simulink model "RL_sus_quarter_sim"  (R2025a)
settings: Solver=FixedStepAuto  StartTime=0.0  StopTime=20  FixedStep=0.001  RelTol=1e-3
model workspace (MAT data in the model file):
  G0 : Simulink.Parameter (value not decoded)
  Q_F : Simulink.Parameter (value not decoded)
  Q_dot_s : Simulink.Parameter (value not decoded)
  Q_dot_s_h : Simulink.Parameter (value not decoded)
  Q_dot_u : Simulink.Parameter (value not decoded)
  Q_flec : Simulink.Parameter (value not decoded)
  Q_flec_t : Simulink.Parameter (value not decoded)
  b_deflec : Simulink.Parameter (value not decoded)
  bump_height : Simulink.Parameter (value not decoded)
  bump_lenth : Simulink.Parameter (value not decoded)
  bump_start : Simulink.Parameter (value not decoded)
  f0 : Simulink.Parameter (value not decoded)
  kt : Simulink.Parameter (value not decoded)
  ms : Simulink.Parameter (value not decoded)
  n0 : Simulink.Parameter (value not decoded)
  n1 : Simulink.Parameter (value not decoded)
  omega_1 : Simulink.Parameter (value not decoded)
  omega_2 : Simulink.Parameter (value not decoded)
  omega_3 : Simulink.Parameter (value not decoded)
  omega_4 : Simulink.Parameter (value not decoded)
  ramp_height : Simulink.Parameter (value not decoded)
  ramp_lenth : Simulink.Parameter (value not decoded)
  ramp_start : Simulink.Parameter (value not decoded)
  sine_amp : Simulink.Parameter (value not decoded)
  sine_freq : Simulink.Parameter (value not decoded)
  u : Simulink.Parameter (value not decoded)
symbols that are objects in the model workspace (value not decoded): b_deflec, bump_height, bump_lenth, bump_start, f0, G0, kt, ms, n0, n1, omega_1, omega_2, omega_3, omega_4, Q_dot_s, Q_dot_s_h, Q_F, Q_flec, Q_flec_t, ramp_height, ramp_lenth, ramp_start, sine_amp, sine_freq
undefined symbols (not defined in the file): Ground, Hook, SH_ADD_new_as_as_xdef
libraries: fl_lib x250, nesl_utility x48, sharedTrackingLibrary x34, dspstat3 x18, simulink x3, deeplib x2, slpidlib x1
(part 4 of 12)

== system RL_sus_quarter_sim/road_profile/origin ==
  Radio Button : RadioButtonGroup  LabelPosition=Hide  SelectedLabel=随机路面  ButtonGroupName=Group
  road_profile : Subsystem
  路面选择 : Constant  Value=3  OutDataTypeStr=int8
  "Road " : Outport
  wires:
  road_profile/1("Road ") -> "Road "/1  "Zr"
  路面选择/1 -> road_profile/1(Road_selection)

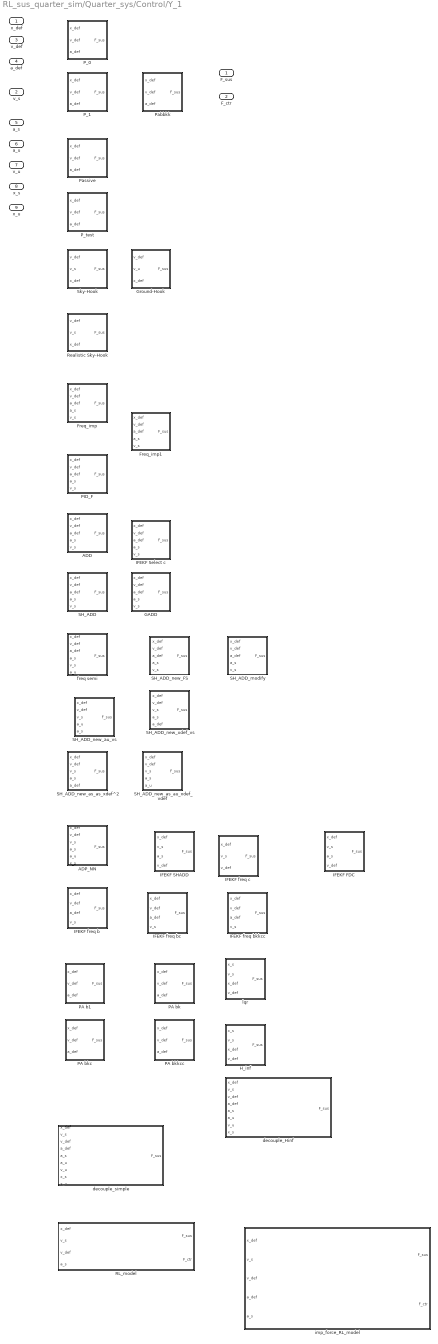
== system RL_sus_quarter_sim/Quarter_sys/Control/Y_1 ==
  x_def : Inport
  v_s : Inport  Port=2
  v_def : Inport  Port=3
  a_def : Inport  Port=4
  a_s : Inport  Port=5
  a_u : Inport  Port=6
  v_u : Inport  Port=7
  x_s : Inport  Port=8
  x_u : Inport  Port=9
  ADD : Subsystem  VariantControl=ADD
  ADP_NN : Subsystem  VariantControl=ADP_nn
  Freq_imp : Subsystem  VariantControl=Freq_Impedance
  Freq_imp1 : Subsystem  VariantControl=Freq_imp1
  GADD : Subsystem  VariantControl=GADD
  Ground-Hook : Subsystem  VariantControl=Ground-Hook
  H_inf : Subsystem  VariantControl=H_inf
  IFEKF FDC : Subsystem  VariantControl=IFEKF FDC
  IFEKF SHADD : Subsystem  VariantControl=IFEKF SHADD
  IFEKF Select c : Subsystem  VariantControl=IFEKF Select imp
  IFEKF freq b : Subsystem  VariantControl=IFEkf freq b
  IFEKF freq bc : Subsystem  VariantControl=IFEKF freq bc
  IFEKF freq bkkcc : Subsystem  VariantControl=IFEKF freq bkkcc
  IFEKF freq c : Subsystem  VariantControl=IFEKF freq c
  PA b1 : Subsystem  VariantControl=PA b1
  PA bk : Subsystem  VariantControl=PA bk
  PA bkc : Subsystem  VariantControl=PA bkc
  PA bkkcc : Subsystem  VariantControl=PA bkkcc
  PID_F : Subsystem  VariantControl=PID_F
  P_0 : Subsystem  VariantControl=p_0
  P_1 : Subsystem  VariantControl=P_1
  P_test : Subsystem  VariantControl=P_test
  Pabbkk : Subsystem  VariantControl=P_2
  Passive : Subsystem  VariantControl=Passive
  RL_model : Subsystem  VariantControl=RL_trained
  Realistic Sky-Hook : Subsystem  VariantControl=Realistic Skyhook
  SH_ADD : Subsystem  VariantControl=SH_ADD
  SH_ADD_modify : Subsystem  VariantControl=SH_ADD_mod
  SH_ADD_new_FS : Subsystem  VariantControl=SH_ADD_new_FS
  SH_ADD_new_as_as_xdef^2 : Subsystem  VariantControl=SH_ADD_new_as_as_xdef^2
  SH_ADD_new_as_au_xdef_vdef : Subsystem  VariantControl=SH_ADD_new_as_au_xdef_vdef
  SH_ADD_new_au_vs : Subsystem  VariantControl=SH_ADD_new_au_vs
  SH_ADD_new_xdef_vs : Subsystem  VariantControl=SH_ADD_new_xdef_vs
  Sky-Hook : Subsystem  VariantControl=SkyHook
  decouple_Hinf : Subsystem  VariantControl=decouple_Hinf
  decouple_simple : Subsystem  VariantControl=decouple_simple
  freq semi : Subsystem  VariantControl=FDC
  imp_force_RL_model : Subsystem  VariantControl=RL_model_imp_force
  lqr : Subsystem  VariantControl=lqr
  F_sus : Outport
  F_ctr : Outport  Port=2

== system RL_sus_quarter_sim/Quarter_sys/Passive/Y_1 ==
  x_def : Inport
  v_def : Inport  Port=2
  a_def : Inport  Port=3
  P_0 : Subsystem  VariantControl=p_0
  P_1 : Subsystem  VariantControl=P_1
  P_test : Subsystem  VariantControl=P_test
  Passive : Subsystem  VariantControl=Passive
  Sky-Hook : Subsystem  VariantControl=SkyHook
  F_sus : Outport

== system RL_sus_quarter_sim/road_profile/origin/road_profile ==
  note: road selection
      | 1 sine
      | 2 chrip
      | 3 random
      | 4 bump
  Road_selection : Inport  OutDataTypeStr=int8  PortDimensions=1
  Bump : Subsystem
  Multiport Switch : MultiPortSwitch  DataPortOrder=Specify indices  Inputs=4  DataPortIndices={1,2,3,4,5}  SaturateOnIntegerOverflow=off  InputSameDT=off
  Ramp : Subsystem
  Random : Subsystem
  Scope{,1..4} (5 alike) : Scope
      Scope settings: ActiveDisplayYMinimum=-0.0025  ActiveDisplayYMaximum=0.0225
      Scope1 settings: ActiveDisplayYMinimum=-0.07212  ActiveDisplayYMaximum=0.08281  DataLoggingVariableName=ScopeData2
      Scope2 settings: ActiveDisplayYMinimum=-0.0025  ActiveDisplayYMaximum=0.0225  DataLoggingVariableName=ScopeData3
      Scope3 settings: ActiveDisplayYMinimum=-0.07918  ActiveDisplayYMaximum=0.12812
      Scope4 settings: ActiveDisplayYMinimum=-0.0025  ActiveDisplayYMaximum=0.0225
  Sine : Subsystem
  chirp : Subsystem
  "Road " : Outport  OutDataTypeStr=double  PortDimensions=1  SampleTime=0  VectorParamsAs1DForOutWhenUnconnected=off
  wires:
  Multiport Switch/1 -> "Road "/1
  Road_selection/1 -> Multiport Switch/1
  chirp/1(Zr) -> Multiport Switch/3, Scope3/1
  Random/1(Zr) -> Scope1/1, Multiport Switch/4
  Sine/1(Out1) -> Multiport Switch/2, Scope/1
  Bump/1(Zr) -> Scope2/1, Multiport Switch/5
  Ramp/1(Zr) -> Scope4/1, Multiport Switch/6

== system RL_sus_quarter_sim/Quarter_sys/Control/Y_1/ADD ==
  x_def : Inport
  v_def : Inport  Port=2
  a_def : Inport  Port=3
  a_s : Inport  Port=4
  v_s : Inport  Port=5
  Add : Sum
  Add1 : Sum
  Constant : Constant  Value=-1
  Constant1 : Constant
  Delta_C : Gain  Gain=500
  Gain : Gain  Gain=-1
  Lmbada_C : Constant  Value=1000
  Product : Product
  Product1 : Product
  Switch : Switch  Criteria=u2 > Threshold  SaturateOnIntegerOverflow=off  InputSameDT=off
  ks : Gain  Gain=-20000
  F_sus : Outport
  wires:
  Constant1/1 -> Switch/1
  a_s/1 -> Product/2
  Lmbada_C/1 -> Add/2
  x_def/1 -> ks/1
  ks/1 -> Add1/2
  Add1/1 -> F_sus/1
  Gain/1 -> Add1/1
  Add/1 -> Product1/2
  Product1/1 -> Gain/1
  Delta_C/1 -> Add/1
  Product/1 -> Switch/2
  Constant/1 -> Switch/3
  Switch/1 -> Delta_C/1
  v_def/1 -> Product/1, Product1/1

== system RL_sus_quarter_sim/Quarter_sys/Control/Y_1/ADP_NN ==
  x_def : Inport
  v_def : Inport  Port=2
  v_s : Inport  Port=3
  a_s : Inport  Port=4
  a_u : Inport  Port=5
  x_s : Inport  Port=6
  ADP_NN_Controller : Subsystem
  Add1 : Sum  Inputs=+++
  Scope : Scope
      settings: ActiveDisplayYMinimum=-1037.91652  ActiveDisplayYMaximum=2906.13276  DataLoggingVariableName=ScopeData5
  cs : Gain  Gain=-1000
  ks : Gain  Gain=-20000
  reference : Subsystem  Variant=on  VariantControlMode=label  VariantControl=skyhook_virtual  LabelModeActiveChoice=zero
  F_sus : Outport
  wires:
  v_s/1 -> reference/2(vs), ADP_NN_Controller/3(vs)
  ks/1 -> Add1/1
  v_def/1 -> ADP_NN_Controller/2(vdef), cs/1
  Add1/1 -> F_sus/1
  cs/1 -> Add1/2
  x_def/1 -> ks/1, ADP_NN_Controller/1(xdef)
  x_s/1 -> reference/1(xs), ADP_NN_Controller/6(xs)
  a_s/1 -> ADP_NN_Controller/4(as)
  a_u/1 -> ADP_NN_Controller/5(au)
  reference/1(xs_ref) -> ADP_NN_Controller/7(xs_ref)
  reference/2(vs_ref) -> ADP_NN_Controller/8(vs_ref)
  ADP_NN_Controller/1(Out1) -> Add1/3, Scope/1

== system RL_sus_quarter_sim/Quarter_sys/Control/Y_1/Freq_imp ==
  x_def : Inport
  v_def : Inport  Port=2
  a_def : Inport  Port=3
  a_s : Inport  Port=4
  v_s : Inport  Port=5
  Add : Sum  Inputs=+-
  Add1 : Sum  Inputs=+-
  Clock : Clock
  Compare To Zero : simulink/Logic and Bit Operations/Compare To Zero  relop=>  OutDataTypeStr=uint8
  Gain : Gain  Gain=2*pi
  Gain1 : Gain  Gain=5
  Low_with_Alpha : Subsystem
  Manual Switch : ManualSwitch  CurrentSetting=0
  Product : Product
  Scope : Scope
      settings: ActiveDisplayYMinimum=-0.125  ActiveDisplayYMaximum=1.125  DataLoggingVariableName=ScopeData17
  Scope1 : Scope
      settings: ActiveDisplayYMinimum=-2.9067065459387251E+17  ActiveDisplayYMaximum=7.876518166218295E+17  DataLoggingVariableName=ScopeData18
  Select_alpha : Constant  Value=5
  Square : Math  Operator=square
  Square1 : Math  Operator=square
  Square2 : Math  Operator=square
  Switch : Switch  Criteria=u2 > Threshold  SaturateOnIntegerOverflow=off  InputSameDT=off
  high_with_Alpha : Subsystem
  F_sus : Outport
  wires:
  v_def/1 -> Low_with_Alpha/1(v_def), high_with_Alpha/1(v_def)
  x_def/1 -> ?
  a_s/1 -> Square/1
  v_s/1 -> Square1/1
  Square1/1 -> Product/1
  Product/1 -> Add/2
  Square/1 -> Add/1
  Manual Switch/1 -> Compare To Zero/1, Scope1/1, Switch/2
  high_with_Alpha/1(F) -> Switch/1
  Low_with_Alpha/1(F) -> Switch/3
  a_def/1 -> Low_with_Alpha/2(a_def), high_with_Alpha/2(a_def)
  Switch/1 -> F_sus/1
  Gain/1 -> Square2/1
  Compare To Zero/1 -> Scope/1
  Square2/1 -> Product/2
  Clock/1 -> Add1/1
  Select_alpha/1 -> Gain1/1, Gain/1
  Gain1/1 -> Add1/2
  Add/1 -> Manual Switch/1
  Add1/1 -> Manual Switch/2

== system RL_sus_quarter_sim/Quarter_sys/Control/Y_1/Freq_imp1 ==
  x_def : Inport
  v_def : Inport  Port=2
  a_def : Inport  Port=3
  a_s : Inport  Port=4
  v_s : Inport  Port=5
  Constant : Constant
  Constant1 : Constant  Value=2
  Low_with_Alpha : Subsystem
  Multiport Switch : MultiPortSwitch  SaturateOnIntegerOverflow=off  InputSameDT=off
  Subsystem : Subsystem
  high_with_Alpha : Subsystem
  F_sus : Outport
  wires:
  Multiport Switch/1 -> F_sus/1
  a_def/1 -> high_with_Alpha/2(a_def), Low_with_Alpha/2(a_def)
  Low_with_Alpha/1(F) -> Multiport Switch/2, Multiport Switch/3
  high_with_Alpha/1(F) -> Multiport Switch/4
  x_def/1 -> ?
  v_def/1 -> high_with_Alpha/1(v_def), Low_with_Alpha/1(v_def)
  Subsystem/1(Select) -> Multiport Switch/1
  a_s/1 -> Subsystem/2(au)
  v_s/1 -> Subsystem/1(vs)
  Constant/1 -> Subsystem/3(alpha1)
  Constant1/1 -> Subsystem/4(alpha2)

== system RL_sus_quarter_sim/Quarter_sys/Control/Y_1/GADD ==
  x_def : Inport
  v_def : Inport  Port=2
  a_def : Inport  Port=3
  a_s : Inport  Port=4
  v_s : Inport  Port=5
  Add : Sum
  Add1 : Sum
  Constant : Constant  Value=-1
  Constant1 : Constant
  Delta_C : Gain  Gain=500
  Gain : Gain  Gain=-1
  Gain1 : Gain  Gain=10
  Lmbada_C : Constant  Value=1000
  Product : Product
  Product1 : Product
  Product2 : Product
  Switch : Switch  Criteria=u2 > Threshold  SaturateOnIntegerOverflow=off  InputSameDT=off
  ks : Gain  Gain=-20000
  F_sus : Outport
  wires:
  v_def/1 -> Product1/1, Product/1
  Switch/1 -> Delta_C/1
  Constant/1 -> Switch/3
  Product/1 -> Switch/2
  Delta_C/1 -> Add/1
  Product1/1 -> Gain/1
  Add/1 -> Product1/2
  Gain/1 -> Add1/1
  Add1/1 -> F_sus/1
  ks/1 -> Add1/2
  x_def/1 -> ks/1
  Lmbada_C/1 -> Add/2
  a_s/1 -> Product2/1
  Constant1/1 -> Switch/1
  v_s/1 -> Gain1/1
  Gain1/1 -> Product2/2
  Product2/1 -> Product/2

== system RL_sus_quarter_sim/Quarter_sys/Control/Y_1/Ground-Hook ==
  v_def : Inport
  v_u : Inport  Port=2
  x_def : Inport  Port=3
  Add : Sum
  Add1 : Sum
  Constant : Constant  Value=-1
  Constant1 : Constant
  Delta_C : Gain  Gain=500
  Gain : Gain  Gain=-1
  Gain1 : Gain  Gain=-1
  Lmbada_C : Constant  Value=1000
  Product : Product
  Product1 : Product
  Switch : Switch  Criteria=u2 > Threshold  SaturateOnIntegerOverflow=off  InputSameDT=off
  ks : Gain  Gain=-20000
  F_sus : Outport
  wires:
  x_def/1 -> ks/1
  ks/1 -> Add1/2
  Add1/1 -> F_sus/1
  Gain/1 -> Add1/1
  Delta_C/1 -> Add/1
  Lmbada_C/1 -> Add/2
  Constant1/1 -> Switch/1
  Constant/1 -> Switch/3
  Product1/1 -> Gain/1
  Switch/1 -> Delta_C/1
  Add/1 -> Product1/2
  v_def/1 -> Product/1, Product1/1
  v_u/1 -> Gain1/1
  Product/1 -> Switch/2
  Gain1/1 -> Product/2

== system RL_sus_quarter_sim/Quarter_sys/Control/Y_1/H_inf ==
  x_s : Inport
  v_s : Inport  Port=2
  x_def : Inport  Port=3
  v_def : Inport  Port=4
  Add : Sum  Inputs=+-
  Add1 : Sum  Inputs=+++
  Add2 : Sum  Inputs=+-
  Gain : Gain
  K : Constant  Value="[-0.0001   -2.8284    6.4278   -0.0257]"
  Mux : Mux
  Product : Product  Multiplication=Matrix(*)
  To Workspace : ToWorkspace  VariableName=F_if_imp  SampleTime=-1
  cs : Gain  Gain=-1000
  ks : Gain  Gain=-20000
  F_sus : Outport
  wires:
  Gain/1 -> To Workspace/1, Add1/3
  Product/1 -> Gain/1
  Mux/1 -> Product/1
  K/1 -> Product/2
  Add2/1 -> Mux/4  "vu"
  Add/1 -> Mux/3  "xu"
  x_def/1 -> Add/2
  cs/1 -> Add1/2  "F_damper"
  ks/1 -> Add1/1
  Add1/1 -> F_sus/1
  x_s/1 -> Mux/1, ks/1, Add/1  "xs"
  v_s/1 -> Mux/2, Add2/1  "vs"
  v_def/1 -> cs/1, Add2/2

== system RL_sus_quarter_sim/Quarter_sys/Control/Y_1/IFEKF FDC ==
  x_def : Inport
  v_s : Inport  Port=2
  a_s : Inport  Port=3
  v_def : Inport  Port=4
  ADD : Subsystem
  Add1 : Sum
  Multiport Switch : MultiPortSwitch  SaturateOnIntegerOverflow=off  InputSameDT=off
  Scope : Scope
      settings: ActiveDisplayYMinimum=0.91612  ActiveDisplayYMaximum=3.17647
  Subsystem : Subsystem
  Subsystem1 : Subsystem
  To Workspace : ToWorkspace  VariableName=FS_result  SampleTime=-1
  ks : Gain  Gain=-20000
  skyhook : Subsystem
  F_sus : Outport
  wires:
  v_def/1 -> Subsystem/2(v_def), ADD/1(v_def), Subsystem1/1(v_def), skyhook/1(v_def)
  a_s/1 -> Subsystem/3(a_s), ADD/2(a_s)
  ks/1 -> Add1/1
  Add1/1 -> F_sus/1
  x_def/1 -> ks/1
  v_s/1 -> Subsystem/1(v_s), skyhook/2(v_s)
  skyhook/1(F_sus1) -> Multiport Switch/2
  ADD/1(Out1) -> Multiport Switch/3
  Multiport Switch/1 -> Add1/2  "F_inerter"
  Subsystem/1(FS_select) -> To Workspace/1, Multiport Switch/1, Scope/1
  Subsystem1/1(Out1) -> Multiport Switch/4

== system RL_sus_quarter_sim/Quarter_sys/Control/Y_1/IFEKF SHADD ==
  x_def : Inport
  v_s : Inport  Port=2
  a_s : Inport  Port=3
  v_def : Inport  Port=4
  ADD : Subsystem
  Add1 : Sum
  Multiport Switch : MultiPortSwitch  Inputs=2  SaturateOnIntegerOverflow=off  InputSameDT=off
  Scope : Scope
      settings: ActiveDisplayYMinimum=0.875  ActiveDisplayYMaximum=2.125
  Subsystem : Subsystem
  ks : Gain  Gain=-20000
  skyhook : Subsystem
  F_sus : Outport
  wires:
  Subsystem/1(FS_select) -> Scope/1, Multiport Switch/1
  Multiport Switch/1 -> Add1/2  "F_inerter"
  ADD/1(Out1) -> Multiport Switch/3
  skyhook/1(F_sus1) -> Multiport Switch/2
  v_s/1 -> skyhook/2(v_s), Subsystem/1(v_s)
  x_def/1 -> ks/1
  Add1/1 -> F_sus/1
  ks/1 -> Add1/1
  a_s/1 -> ADD/2(a_s)
  v_def/1 -> skyhook/1(v_def), ADD/1(v_def)

== system RL_sus_quarter_sim/Quarter_sys/Control/Y_1/IFEKF Select c ==
  x_def : Inport
  v_def : Inport  Port=2
  a_def : Inport  Port=3
  a_s : Inport  Port=4
  v_s : Inport  Port=5
  Add : Sum
  Scope : Scope
      settings: ActiveDisplayYMinimum=0.75  ActiveDisplayYMaximum=3.25  DataLoggingVariableName=ScopeData3
  Subsystem : Subsystem
  Subsystem2 : Subsystem  Variant=on  VariantControlMode=label  VariantControl=Subsystem2  LabelModeActiveChoice=constant
  ks : Gain  Gain=-20000
  F_sus : Outport
  wires:
  v_s/1 -> Subsystem/1(In1), Subsystem2/3(v_s)
  Subsystem/1(FS_select) -> Scope/1, Subsystem2/1(sig select)
  Add/1 -> F_sus/1
  ks/1 -> Add/2  "F Spring"
  x_def/1 -> ks/1
  v_def/1 -> Subsystem2/2(v_def)
  a_s/1 -> Subsystem2/4(a_s)
  Subsystem2/1(F_damper) -> Add/1

== system RL_sus_quarter_sim/Quarter_sys/Control/Y_1/IFEKF freq b ==
  x_def : Inport
  v_def : Inport  Port=2
  a_def : Inport  Port=3
  v_s : Inport  Port=4
  Add1 : Sum  Inputs=+++
  Multiport Switch : MultiPortSwitch  SaturateOnIntegerOverflow=off  InputSameDT=off
  Subsystem : Subsystem
  cs : Gain  Gain=-1000
  ks : Gain  Gain=-20000
  large b : Subsystem
  mid b : Subsystem
  small  b : Subsystem
  F_sus : Outport
  wires:
  ks/1 -> Add1/1
  v_def/1 -> cs/1
  Add1/1 -> F_sus/1
  cs/1 -> Add1/2
  x_def/1 -> ks/1
  v_s/1 -> Subsystem/1(v_s)
  large b/1(F_sus1) -> Multiport Switch/4
  small  b/1(Out1) -> Multiport Switch/2
  a_def/1 -> mid b/1(a_def), small  b/1(a_def), large b/1(a_def)
  Multiport Switch/1 -> Add1/3  "F_inerter"
  Subsystem/1(FS_select) -> Multiport Switch/1
  mid b/1(Out1) -> Multiport Switch/3

== system RL_sus_quarter_sim/Quarter_sys/Control/Y_1/IFEKF freq bc ==
  x_def : Inport
  v_def : Inport  Port=2
  a_def : Inport  Port=3
  v_s : Inport  Port=4
  Add1 : Sum  Inputs=+++
  Multiport Switch : MultiPortSwitch  SaturateOnIntegerOverflow=off  InputSameDT=off
  Multiport Switch1 : MultiPortSwitch  Inputs=2  SaturateOnIntegerOverflow=off  InputSameDT=off
  Subsystem : Subsystem
  ks : Gain  Gain=-20000
  large C : Subsystem
  large b : Subsystem
  mid b : Subsystem
  small  b : Subsystem
  small C : Subsystem
  F_sus : Outport
  wires:
  mid b/1(Out1) -> Multiport Switch/3
  Subsystem/1(FS_select b) -> Multiport Switch/1
  Multiport Switch/1 -> Add1/3  "F_inerter"
  a_def/1 -> large b/1(a_def), small  b/1(a_def), mid b/1(a_def)
  small  b/1(Out1) -> Multiport Switch/2
  large b/1(F_sus1) -> Multiport Switch/4
  v_s/1 -> Subsystem/1(v_s)
  x_def/1 -> ks/1
  Add1/1 -> F_sus/1
  ks/1 -> Add1/1
  large C/1(F_sus1) -> Multiport Switch1/3
  small C/1(Out1) -> Multiport Switch1/2
  v_def/1 -> small C/1(v_def), large C/1(v_def)
  Multiport Switch1/1 -> Add1/2  "F_damper"
  Subsystem/2(FS_select c) -> Multiport Switch1/1

== system RL_sus_quarter_sim/Quarter_sys/Control/Y_1/IFEKF freq bkkcc ==
  x_def : Inport
  v_def : Inport  Port=2
  a_def : Inport  Port=3
  v_s : Inport  Port=4
  Add1 : Sum  Inputs=+++
  Subsystem : Subsystem
  Subsystem1 : Subsystem
  To Workspace : ToWorkspace  VariableName=F_if_imp  SampleTime=-1
  Transfer Fcn : TransferFcn  Numerator=[1000*10 0]  Denominator=[10 1000]
  bkkcc : Subsystem
  cs : Gain  Gain=-1000
  ks : Gain  Gain=-20000
  F_sus : Outport
  wires:
  cs/1 -> Add1/2  "F_damper"
  ks/1 -> Add1/1
  Add1/1 -> F_sus/1
  x_def/1 -> ks/1, Subsystem1/2(input0), bkkcc/2(x_def)
  v_s/1 -> Subsystem/1(v_s)
  a_def/1 -> Subsystem1/1(input1), bkkcc/3(a_def)
  v_def/1 -> Transfer Fcn/1, bkkcc/1(v_def), cs/1
  Subsystem1/1(output) -> ?
  bkkcc/1(F_bkkcc) -> To Workspace/1, Add1/3
  Subsystem/1(Out1) -> bkkcc/4(param_ctr)

== system RL_sus_quarter_sim/Quarter_sys/Control/Y_1/IFEKF freq c ==
  x_def : Inport
  v_s : Inport  Port=2
  v_def : Inport  Port=3
  Add1 : Sum
  Large C : Subsystem
  Mid C : Subsystem
  Multiport Switch : MultiPortSwitch  Inputs=4  SaturateOnIntegerOverflow=off  InputSameDT=off
  Scope : Scope
      settings: ActiveDisplayYMinimum=0.625  ActiveDisplayYMaximum=4.375
  Small C : Subsystem
  Subsystem : Subsystem
  ks : Gain  Gain=-20000
  F_sus : Outport
  wires:
  v_def/1 -> Large C/1(v_def), Mid C/1(v_def), Small C/1(v_def)
  ks/1 -> Add1/1
  Add1/1 -> F_sus/1
  x_def/1 -> ks/1
  v_s/1 -> Subsystem/1(v_s)
  Multiport Switch/1 -> Add1/2  "F_inerter"
  Subsystem/1(FS_select) -> Scope/1, Multiport Switch/1
  Small C/1(Out1) -> Multiport Switch/3
  Large C/1(Out1) -> Multiport Switch/4, Multiport Switch/2
  Mid C/1(Out1) -> Multiport Switch/5

== system RL_sus_quarter_sim/Quarter_sys/Control/Y_1/PA b1 ==
  x_def : Inport
  v_def : Inport  Port=2
  a_def : Inport  Port=3
  Add1 : Sum  Inputs=+++
  Constant : Constant  Value=10
  Gain : Gain  Gain=-1
  Product : Product
  cs : Gain  Gain=-1000
  ks : Gain  Gain=-20000
  F_sus : Outport
  wires:
  x_def/1 -> ks/1
  cs/1 -> Add1/2
  Add1/1 -> F_sus/1
  v_def/1 -> cs/1
  ks/1 -> Add1/1
  Product/1 -> Gain/1
  a_def/1 -> Product/1
  Gain/1 -> Add1/3
  Constant/1 -> Product/2

== system RL_sus_quarter_sim/Quarter_sys/Control/Y_1/PA bk ==
  x_def : Inport
  v_def : Inport  Port=2
  a_def : Inport  Port=3
  Add1 : Sum  Inputs=+++
  Subsystem : Subsystem
  cs : Gain  Gain=-1000
  ks : Gain  Gain=-20000
  F_sus : Outport
  wires:
  ks/1 -> Add1/1
  Add1/1 -> F_sus/1
  cs/1 -> Add1/2
  x_def/1 -> ks/1
  v_def/1 -> Subsystem/1(input0), cs/1
  a_def/1 -> Subsystem/2(input1)
  Subsystem/1(output) -> Add1/3

== system RL_sus_quarter_sim/Quarter_sys/Control/Y_1/PA bkc ==
  x_def : Inport
  v_def : Inport  Port=2
  a_def : Inport  Port=3
  Add1 : Sum  Inputs=+++
  Subsystem : Subsystem
  cs : Gain  Gain=-1000
  ks : Gain  Gain=-20000
  F_sus : Outport
  wires:
  Subsystem/1(output) -> Add1/3
  a_def/1 -> Subsystem/2(input1)
  v_def/1 -> cs/1, Subsystem/1(input0)
  x_def/1 -> ks/1
  cs/1 -> Add1/2
  Add1/1 -> F_sus/1
  ks/1 -> Add1/1

== system RL_sus_quarter_sim/Quarter_sys/Control/Y_1/PA bkkcc ==
  x_def : Inport
  v_def : Inport  Port=2
  a_def : Inport  Port=3
  Add1 : Sum  Inputs=+++
  Subsystem : Subsystem
  cs : Gain  Gain=-500
  ks : Gain  Gain=-30000
  F_sus : Outport
  wires:
  ks/1 -> Add1/1
  Add1/1 -> F_sus/1
  cs/1 -> Add1/2
  x_def/1 -> ks/1
  v_def/1 -> Subsystem/1(input0), cs/1
  a_def/1 -> Subsystem/2(input1)
  Subsystem/1(output) -> Add1/3

== system RL_sus_quarter_sim/Quarter_sys/Control/Y_1/PID_F ==
  x_def : Inport
  v_def : Inport  Port=2
  a_def : Inport  Port=3
  a_s : Inport  Port=4
  v_s : Inport  Port=5
  Add : Sum
  Add1 : Sum  Inputs=+-
  Add2 : Sum
  Constant : Constant  Value=5
  Constant1 : Constant
  Gain : Gain  Gain=-2000
  Gain1 : Gain  Gain=-20000
  Memory : Memory
  PID Controller : slpidlib/PID Controller  Controller=PID  Form=Parallel  TimeDomain=Continuous-time  UseExternalTs=off  SampleTime=-1  IntegratorMethod=Forward Euler  FilterMethod=Forward Euler  ControllerParametersSource=internal  P=1  I=0.0001  UseKiTs=off  D=0  UseExternalDerivativeSource=off  N=100  UseFilter=on  TunerSelectOption=Transfer Function Based (PID Tuner App)  InitialConditionSource=internal  InitialConditionForIntegrator=0  InitialConditionForFilter=0  DifferentiatorICPrevScaledInput=0  ExternalReset=none  TrackingMode=off  Kt=1  LimitOutput=off  SatLimitsSource=internal  UpperSaturationLimit=inf  LowerSaturationLimit=-inf  LinearizeAsGain=on  AntiWindupMode=none  Kb=1  LimitIntegrator=off  UpperIntegratorSaturationLimit=inf  LowerIntegratorSaturationLimit=-inf  POutMin=[]  POutMax=[]  IOutMin=[]  IOutMax=[]  DOutMin=[]  DOutMax=[]  NOutMin=[]  NOutMax=[]  SumOutMin=[]  SumOutMax=[]  SaturationOutMin=[]  SaturationOutMax=[]  PParamMin=[]  PParamMax=[]  IParamMin=[]  IParamMax=[]  DParamMin=[]  DParamMax=[]  NParamMin=[]  NParamMax=[]  KbParamMin=[]  KbParamMax=[]  KtParamMin=[]  KtParamMax=[]  KbOutMin=[]  KbOutMax=[]  KtOutMin=[]  KtOutMax=[]  IntegratorOutMin=[]  IntegratorOutMax=[]  FilterOutMin=[]  FilterOutMax=[]  SumI1OutMin=[]  SumI1OutMax=[]  SumI2OutMin=[]  SumI2OutMax=[]  SumI3OutMin=[]  SumI3OutMax=[]  SumI4OutMin=[]  SumI4OutMax=[]  SumDOutMin=[]  SumDOutMax=[]  DifferentiatorOutMin=[]  DifferentiatorOutMax=[]  FilterDiffOutCoefMin=[]  FilterDiffOutCoefMax=[]  ReciprocalOutMin=[]  ReciprocalOutMax=[]  SumDenOutMin=[]  SumDenOutMax=[]  SumNumOutMin=[]  SumNumOutMax=[]  DivideOutMin=[]  DivideOutMax=[]  UdiffTsProdOutMin=[]  UdiffTsProdOutMax=[]  NTsProdOutMin=[]  NTsProdOutMax=[]  UintegralTsProdOutMin=[]  UintegralTsProdOutMax=[]  UngainTsProdOutMin=[]  UngainTsProdOutMax=[]  ClampingZeroOutDataTypeStr=Inherit: Inherit via back propagation  ClampingZeroOutMin=[]  ClampingZeroOutMax=[]  FilterDenConstantOutDataTypeStr=Inherit: Inherit via back propagation  FilterDenConstantOutMin=[]  FilterDenConstantOutMax=[]  PCopyOutDataTypeStr=Inherit: Inherit via back propagation  PCopyOutMin=[]  PCopyOutMax=[]  NCopyOutDataTypeStr=Inherit: Inherit via back propagation  NCopyOutMin=[]  NCopyOutMax=[]  IntegratorContinuousStateAttributes=''  IntegratorStateMustResolveToSignalObject=off  IntegratorRTWStateStorageClass=Auto  FilterContinuousStateAttributes=''  FilterStateMustResolveToSignalObject=off  FilterRTWStateStorageClass=Auto  ParallelPVariant=InternalParameters  IdealPVariant=Disabled  IVariant=InternalParameters  DVariant=InternalParameters  IntegratorVariant=Continuous  SatVariant=Disabled  AWVariant=Passthrough  PCopyVariant=Disabled  TRVariant=Disabled  FdbkBlocksVariant=Forward  IdealPFdbkVariant=Disabled  SatFdbkVariant=Disabled  DerivativeFilterVariant=ContFilter  NVariant=InternalParameters  NCopyVariant=Disabled  FilterICVariant=InternalICsFilter  IntegratorICVariant=InternalICs  ExternalResetVariant=Disabled  TRSumVariant=Passthrough  SumFdbkVariant=Disabled  SumVariant=Sum_PID  TsampFilterVariant=InternalTs  TsampNgainVariant=Passthrough  TsampIntegralVariant=Disabled_SignalSpec  ExternalSaturationOutDataTypeStr=Inherit: Same as second input  DerivativeSourceVariant=ErrorSignal  PreIntVariant=InternalPreInt
  Product : Product
  Scope : Scope  NumInputPorts=2
      settings: ActiveDisplayYMinimum=-1305.7038  ActiveDisplayYMaximum=1706.20222
  F_sus : Outport
  wires:
  PID Controller/1 -> Add2/1
  Product/1 -> Scope/1
  v_def/1 -> Gain/1
  x_def/1 -> Gain1/1
  Add/1 -> Memory/1, F_sus/1, Add1/2, Scope/2
  Memory/1 -> Add1/1  "sensor"
  Add1/1 -> PID Controller/1
  Add2/1 -> Product/1
  Constant/1 -> Add2/2
  Constant1/1 -> Product/2
  Gain/1 -> Add/2
  Gain1/1 -> Add/1

== system RL_sus_quarter_sim/Quarter_sys/Control/Y_1/P_0 ==
  x_def : Inport
  v_def : Inport  Port=2
  a_def : Inport  Port=3
  Add1 : Sum
  Ideal Force Sensor : fl_lib/Mechanical/Mechanical Sensors/Ideal Force Sensor
  Ideal Translational Velocity Source : fl_lib/Mechanical/Mechanical Sources/Ideal Translational Velocity Source
  Mechanical Translational Reference : fl_lib/Mechanical/Translational Elements/Mechanical Translational Reference
  Mechanical Translational Reference1 : fl_lib/Mechanical/Translational Elements/Mechanical Translational Reference
  PS-Simulink Converter : nesl_utility/PS-Simulink Converter  PhysicalDomain=network_engine_domain  SubClassName=ps_output  LeftPortType=input  RightPortType=output  PseudoPeriodic=off  Frequencies=[]  VectorFormat=inherit  Unit=inherit  AffineConversion=off
  Scope : Scope  NumInputPorts=2
      settings: ActiveDisplayYMinimum=-2784.63973  ActiveDisplayYMaximum=3155.95467
  Simulink-PS Converter : nesl_utility/Simulink-PS Converter  PhysicalDomain=network_engine_domain  SubClassName=ps_input  LeftPortType=input  RightPortType=output  PseudoPeriodic=off  Frequencies=[]  NoiseDistribution=none  NoiseParameters=[]  Unit=1  AffineConversion=off  FilteringAndDerivatives=provide  SimscapeFilterOrder=1  InputFilterTimeConstant=0.001  UdotUserProvided=0
  Solver Configuration : nesl_utility/Solver Configuration  PhysicalDomain=network_engine_domain  SubClassName=solver  LeftPortType=input  RightPortType=generic  Tones=[]  Harmonics=[]  SimulateNoise=off  Profile=off  UseLocalSampling=off  EnableSwitchedLinearOptims=on  FrequencyDomain=off  UseCCode=off  RelTol=0.001  AbsTol=0.001  MinStep=1e-09  ToWorkspace=off  RevertToSquareIcSolve=off  NumHomotopyIterations=100  PhasorMode=off  PhasorModeNumHarmonics=1  ConsistencySolver=NEWTON_XTOL_AFTER_FTOL  IndexReductionMethod=DerivativeReplacement  DoDC=off  ResidualTolerance=1e-09  ConsistencyTolSource=GLOBAL  ConsistencyAbsTol=0.001  ConsistencyRelTol=0.001  ConsistencyTolFactor=0.001  UseLocalSolver=off  LocalSolverChoice=NE_BACKWARD_EULER_ADVANCER  ResolveIndetEquations=on  FunctionEvalNumThread=1  LocalSolverSampleTime=0.001  DoFixedCost=off  MaxNonlinIter=3  MaxModeIter=2  ComputeImpulses=off  ImpulseIterations=2  LinearAlgebra=auto  LinearAlgebraNumThread=0  EquationFormulation=NE_TIME_EF  DelaysMemoryBudget=1024  AutomaticFiltering=on  FilteringTimeConstant=0.001  PartitionStorageMethod=AS_NEEDED  PartitionMemoryBudget=1024  PartitionMethod=ROBUST  MultibodyUseLocalSolver=off  MultibodyLocalSolverChoice=ODE1  MultibodyLocalSolverSampleTime=0.001
  Subsystem : Subsystem  Variant=on  VariantControlMode=label  VariantControl=Subsystem  LabelModeActiveChoice=p0_k6
  cs : Gain  Gain=-2000
  ks : Gain  Gain=-200000
  F_sus : Outport
  wires:
  PS-Simulink Converter/1 -> Scope/1, F_sus/1
  v_def/1 -> cs/1, Simulink-PS Converter/1
  ks/1 -> Add1/1
  cs/1 -> Add1/2
  x_def/1 -> ks/1
  connections:
  Subsystem/RConn1 -- Ideal Force Sensor/LConn1
  Subsystem/LConn1 -- Ideal Translational Velocity Source/RConn2
  PS-Simulink Converter/LConn1 -- Ideal Force Sensor/RConn2
  Ideal Force Sensor/RConn1 -- Mechanical Translational Reference/LConn1
  Simulink-PS Converter/RConn1 -- Ideal Translational Velocity Source/RConn1
  Solver Configuration/RConn1 -- Mechanical Translational Reference1/LConn1 -- Ideal Translational Velocity Source/LConn1

== system RL_sus_quarter_sim/Quarter_sys/Control/Y_1/P_1 ==
  x_def : Inport
  v_def : Inport  Port=2
  a_def : Inport  Port=3
  Add1 : Sum
  Ideal Force Sensor : fl_lib/Mechanical/Mechanical Sensors/Ideal Force Sensor
  Ideal Translational Velocity Source : fl_lib/Mechanical/Mechanical Sources/Ideal Translational Velocity Source
  Mechanical Translational Reference : fl_lib/Mechanical/Translational Elements/Mechanical Translational Reference
  Mechanical Translational Reference1 : fl_lib/Mechanical/Translational Elements/Mechanical Translational Reference
  PS-Simulink Converter : nesl_utility/PS-Simulink Converter  PhysicalDomain=network_engine_domain  SubClassName=ps_output  LeftPortType=input  RightPortType=output  PseudoPeriodic=off  Frequencies=[]  VectorFormat=inherit  Unit=inherit  AffineConversion=off
  Scope : Scope  NumInputPorts=2
      settings: ActiveDisplayYMinimum=-2784.63973  ActiveDisplayYMaximum=3155.95467
  Simulink-PS Converter : nesl_utility/Simulink-PS Converter  PhysicalDomain=network_engine_domain  SubClassName=ps_input  LeftPortType=input  RightPortType=output  PseudoPeriodic=off  Frequencies=[]  NoiseDistribution=none  NoiseParameters=[]  Unit=1  AffineConversion=off  FilteringAndDerivatives=provide  SimscapeFilterOrder=1  InputFilterTimeConstant=0.001  UdotUserProvided=1
  Solver Configuration : nesl_utility/Solver Configuration  PhysicalDomain=network_engine_domain  SubClassName=solver  LeftPortType=input  RightPortType=generic  Tones=[]  Harmonics=[]  SimulateNoise=off  Profile=off  UseLocalSampling=off  EnableSwitchedLinearOptims=on  FrequencyDomain=off  UseCCode=off  RelTol=0.001  AbsTol=0.001  MinStep=1e-09  ToWorkspace=off  RevertToSquareIcSolve=off  NumHomotopyIterations=100  PhasorMode=off  PhasorModeNumHarmonics=1  ConsistencySolver=NEWTON_XTOL_AFTER_FTOL  IndexReductionMethod=DerivativeReplacement  DoDC=off  ResidualTolerance=1e-09  ConsistencyTolSource=GLOBAL  ConsistencyAbsTol=0.001  ConsistencyRelTol=0.001  ConsistencyTolFactor=0.001  UseLocalSolver=off  LocalSolverChoice=NE_BACKWARD_EULER_ADVANCER  ResolveIndetEquations=on  FunctionEvalNumThread=1  LocalSolverSampleTime=0.001  DoFixedCost=off  MaxNonlinIter=3  MaxModeIter=2  ComputeImpulses=off  ImpulseIterations=2  LinearAlgebra=auto  LinearAlgebraNumThread=0  EquationFormulation=NE_TIME_EF  DelaysMemoryBudget=1024  AutomaticFiltering=on  FilteringTimeConstant=0.001  PartitionStorageMethod=AS_NEEDED  PartitionMemoryBudget=1024  PartitionMethod=ROBUST  MultibodyUseLocalSolver=off  MultibodyLocalSolverChoice=ODE1  MultibodyLocalSolverSampleTime=0.001
  Subsystem : Subsystem  Variant=on  VariantControlMode=label  VariantControl=Subsystem  LabelModeActiveChoice=p1_k1
  cs : Gain  Gain=-2000
  ks : Gain  Gain=-200000
  F_sus : Outport
  wires:
  a_def/1 -> Simulink-PS Converter/2
  x_def/1 -> ks/1
  cs/1 -> Add1/2
  ks/1 -> Add1/1
  v_def/1 -> Simulink-PS Converter/1, cs/1
  PS-Simulink Converter/1 -> Scope/1, F_sus/1
  connections:
  Ideal Translational Velocity Source/LConn1 -- Mechanical Translational Reference1/LConn1 -- Solver Configuration/RConn1
  Simulink-PS Converter/RConn1 -- Ideal Translational Velocity Source/RConn1
  Ideal Force Sensor/RConn1 -- Mechanical Translational Reference/LConn1
  PS-Simulink Converter/LConn1 -- Ideal Force Sensor/RConn2
  Subsystem/LConn1 -- Ideal Translational Velocity Source/RConn2
  Subsystem/RConn1 -- Ideal Force Sensor/LConn1

== system RL_sus_quarter_sim/Quarter_sys/Control/Y_1/P_test ==
  x_def : Inport
  v_def : Inport  Port=2
  a_def : Inport  Port=3
  Add : Sum  Inputs=+-
  Add1 : Sum
  Ideal Force Sensor : fl_lib/Mechanical/Mechanical Sensors/Ideal Force Sensor
  Ideal Translational Velocity Source : fl_lib/Mechanical/Mechanical Sources/Ideal Translational Velocity Source
  Integrator : Integrator
  Mechanical Translational Reference : fl_lib/Mechanical/Translational Elements/Mechanical Translational Reference
  Mechanical Translational Reference1 : fl_lib/Mechanical/Translational Elements/Mechanical Translational Reference
  PS-Simulink Converter : nesl_utility/PS-Simulink Converter  PhysicalDomain=network_engine_domain  SubClassName=ps_output  LeftPortType=input  RightPortType=output  PseudoPeriodic=off  Frequencies=[]  VectorFormat=inherit  Unit=inherit  AffineConversion=off
  Scope : Scope  NumInputPorts=2
      settings: ActiveDisplayYMinimum=-1294.98501  ActiveDisplayYMaximum=1379.176
  Simulink-PS Converter : nesl_utility/Simulink-PS Converter  PhysicalDomain=network_engine_domain  SubClassName=ps_input  LeftPortType=input  RightPortType=output  PseudoPeriodic=off  Frequencies=[]  NoiseDistribution=none  NoiseParameters=[]  Unit=1  AffineConversion=off  FilteringAndDerivatives=provide  SimscapeFilterOrder=1  InputFilterTimeConstant=0.001  UdotUserProvided=1
  Solver Configuration : nesl_utility/Solver Configuration  PhysicalDomain=network_engine_domain  SubClassName=solver  LeftPortType=input  RightPortType=generic  Tones=[]  Harmonics=[]  SimulateNoise=off  Profile=off  UseLocalSampling=off  EnableSwitchedLinearOptims=on  FrequencyDomain=off  UseCCode=off  RelTol=0.001  AbsTol=0.001  MinStep=1e-09  ToWorkspace=off  RevertToSquareIcSolve=off  NumHomotopyIterations=100  PhasorMode=off  PhasorModeNumHarmonics=1  ConsistencySolver=NEWTON_XTOL_AFTER_FTOL  IndexReductionMethod=DerivativeReplacement  DoDC=off  ResidualTolerance=1e-09  ConsistencyTolSource=GLOBAL  ConsistencyAbsTol=0.001  ConsistencyRelTol=0.001  ConsistencyTolFactor=0.001  UseLocalSolver=off  LocalSolverChoice=NE_BACKWARD_EULER_ADVANCER  ResolveIndetEquations=on  FunctionEvalNumThread=1  LocalSolverSampleTime=0.001  DoFixedCost=off  MaxNonlinIter=3  MaxModeIter=2  ComputeImpulses=off  ImpulseIterations=2  LinearAlgebra=auto  LinearAlgebraNumThread=0  EquationFormulation=NE_TIME_EF  DelaysMemoryBudget=1024  AutomaticFiltering=on  FilteringTimeConstant=0.001  PartitionStorageMethod=AS_NEEDED  PartitionMemoryBudget=1024  PartitionMethod=ROBUST  MultibodyUseLocalSolver=off  MultibodyLocalSolverChoice=ODE1  MultibodyLocalSolverSampleTime=0.001
  Subsystem : Subsystem  Commented=on  Variant=on  VariantControlMode=label  VariantControl=Subsystem  LabelModeActiveChoice=p1_k3
  Translational Damper : fl_lib/Mechanical/Translational Elements/Translational Damper  D=2000 N*s/m  v_specify=off  v_priority=None  v=0 m/s  v_nominal_specify=off  v_nominal_value=1  v_nominal_unit=m/s  f_specify=off  f_priority=None  f=0 N  f_nominal_specify=off  f_nominal_value=1  f_nominal_unit=N
  Translational Spring1 : fl_lib/Mechanical/Translational Elements/Translational Spring  spr_rate=200000 N/m  v_specify=off  v_priority=None  v=0 m/s  v_nominal_specify=off  v_nominal_value=1  v_nominal_unit=m/s  f_specify=off  f_priority=None  f=0 N  f_nominal_specify=off  f_nominal_value=1  f_nominal_unit=N  x_specify=off  x_priority=High  x=0 m  x_nominal_specify=off  x_nominal_value=1  x_nominal_unit=m
  Translational Spring2 : fl_lib/Mechanical/Translational Elements/Translational Spring  spr_rate=20000 N/m  v_specify=off  v_priority=None  v=0 m/s  v_nominal_specify=off  v_nominal_value=1  v_nominal_unit=m/s  f_specify=off  f_priority=None  f=0 N  f_nominal_specify=off  f_nominal_value=1  f_nominal_unit=N  x_specify=off  x_priority=High  x=0 m  x_nominal_specify=off  x_nominal_value=1  x_nominal_unit=m
  cs : Gain  Gain=-2000
  cs1 : Gain  Gain=20000/2000
  ks : Gain  Gain=-20000
  ks1 : Gain  Gain=-20000
  F_sus : Outport
  wires:
  cs1/1 -> Add/2
  Add/1 -> Integrator/1
  ks1/1 -> Add/1
  Integrator/1 -> Scope/2, cs1/1
  PS-Simulink Converter/1 -> F_sus/1, Scope/1
  v_def/1 -> cs/1, Simulink-PS Converter/1, ks1/1
  ks/1 -> Add1/1
  cs/1 -> Add1/2
  x_def/1 -> ks/1
  a_def/1 -> Simulink-PS Converter/2
  connections:
  Translational Spring1/LConn1 -- Translational Damper/RConn1
  Translational Spring2/RConn1 -- Translational Spring1/RConn1 -- Subsystem/RConn1 -- Ideal Force Sensor/LConn1
  Translational Spring2/LConn1 -- Translational Damper/LConn1 -- Subsystem/LConn1 -- Ideal Translational Velocity Source/RConn2
  PS-Simulink Converter/LConn1 -- Ideal Force Sensor/RConn2
  Ideal Force Sensor/RConn1 -- Mechanical Translational Reference/LConn1
  Simulink-PS Converter/RConn1 -- Ideal Translational Velocity Source/RConn1
  Solver Configuration/RConn1 -- Mechanical Translational Reference1/LConn1 -- Ideal Translational Velocity Source/LConn1

== system RL_sus_quarter_sim/Quarter_sys/Control/Y_1/Pabbkk ==
  x_def : Inport
  v_def : Inport  Port=2
  a_def : Inport  Port=3
  Add1 : Sum
  Ideal Force Sensor : fl_lib/Mechanical/Mechanical Sensors/Ideal Force Sensor
  Ideal Translational Velocity Source : fl_lib/Mechanical/Mechanical Sources/Ideal Translational Velocity Source
  Mechanical Translational Reference : fl_lib/Mechanical/Translational Elements/Mechanical Translational Reference
  Mechanical Translational Reference1 : fl_lib/Mechanical/Translational Elements/Mechanical Translational Reference
  PS-Simulink Converter : nesl_utility/PS-Simulink Converter  PhysicalDomain=network_engine_domain  SubClassName=ps_output  LeftPortType=input  RightPortType=output  PseudoPeriodic=off  Frequencies=[]  VectorFormat=inherit  Unit=inherit  AffineConversion=off
  Scope : Scope  NumInputPorts=2
      settings: ActiveDisplayYMinimum=-2784.63973  ActiveDisplayYMaximum=3155.95467
  Simulink-PS Converter : nesl_utility/Simulink-PS Converter  PhysicalDomain=network_engine_domain  SubClassName=ps_input  LeftPortType=input  RightPortType=output  PseudoPeriodic=off  Frequencies=[]  NoiseDistribution=none  NoiseParameters=[]  Unit=1  AffineConversion=off  FilteringAndDerivatives=provide  SimscapeFilterOrder=1  InputFilterTimeConstant=0.001  UdotUserProvided=1
  Solver Configuration : nesl_utility/Solver Configuration  PhysicalDomain=network_engine_domain  SubClassName=solver  LeftPortType=input  RightPortType=generic  Tones=[]  Harmonics=[]  SimulateNoise=off  Profile=off  UseLocalSampling=off  EnableSwitchedLinearOptims=on  FrequencyDomain=off  UseCCode=off  RelTol=0.001  AbsTol=0.001  MinStep=1e-09  ToWorkspace=off  RevertToSquareIcSolve=off  NumHomotopyIterations=100  PhasorMode=off  PhasorModeNumHarmonics=1  ConsistencySolver=NEWTON_XTOL_AFTER_FTOL  IndexReductionMethod=DerivativeReplacement  DoDC=off  ResidualTolerance=1e-09  ConsistencyTolSource=GLOBAL  ConsistencyAbsTol=0.001  ConsistencyRelTol=0.001  ConsistencyTolFactor=0.001  UseLocalSolver=off  LocalSolverChoice=NE_BACKWARD_EULER_ADVANCER  ResolveIndetEquations=on  FunctionEvalNumThread=1  LocalSolverSampleTime=0.001  DoFixedCost=off  MaxNonlinIter=3  MaxModeIter=2  ComputeImpulses=off  ImpulseIterations=2  LinearAlgebra=auto  LinearAlgebraNumThread=0  EquationFormulation=NE_TIME_EF  DelaysMemoryBudget=1024  AutomaticFiltering=on  FilteringTimeConstant=0.001  PartitionStorageMethod=AS_NEEDED  PartitionMemoryBudget=1024  PartitionMethod=ROBUST  MultibodyUseLocalSolver=off  MultibodyLocalSolverChoice=ODE1  MultibodyLocalSolverSampleTime=0.001
  Subsystem : Subsystem  Variant=on  VariantControlMode=label  VariantControl=Subsystem  LabelModeActiveChoice=p1_k1
  cs : Gain  Gain=-2000
  ks : Gain  Gain=-200000
  F_sus : Outport
  wires:
  PS-Simulink Converter/1 -> F_sus/1, Scope/1
  v_def/1 -> cs/1, Simulink-PS Converter/1
  ks/1 -> Add1/1
  cs/1 -> Add1/2
  x_def/1 -> ks/1
  a_def/1 -> Simulink-PS Converter/2
  connections:
  Subsystem/RConn1 -- Ideal Force Sensor/LConn1
  Subsystem/LConn1 -- Ideal Translational Velocity Source/RConn2
  PS-Simulink Converter/LConn1 -- Ideal Force Sensor/RConn2
  Ideal Force Sensor/RConn1 -- Mechanical Translational Reference/LConn1
  Simulink-PS Converter/RConn1 -- Ideal Translational Velocity Source/RConn1
  Solver Configuration/RConn1 -- Mechanical Translational Reference1/LConn1 -- Ideal Translational Velocity Source/LConn1

== system RL_sus_quarter_sim/Quarter_sys/Control/Y_1/Passive ==
  x_def : Inport
  v_def : Inport  Port=2
  a_def : Inport  Port=3
  Add1 : Sum
  cs : Gain  Gain=-1000
  ks : Gain  Gain=-20000
  F_sus : Outport
  wires:
  x_def/1 -> ks/1
  cs/1 -> Add1/2
  ks/1 -> Add1/1
  v_def/1 -> cs/1
  Add1/1 -> F_sus/1

== system RL_sus_quarter_sim/Quarter_sys/Control/Y_1/RL_model ==
  x_def : Inport
  v_s : Inport  Port=2
  v_def : Inport  Port=3
  a_s : Inport  Port=4
  Add : Sum
  Add1 : Sum
  Constant : Constant  Value=0.5
  Constant1 : Constant  Value=0.5
  Constant2 : Constant  Value=0.5
  Gain : Gain  Gain=1000
  Gain1 : Gain  Gain=1/5
  Gain2 : Gain  Gain=1/0.3
  Gain3 : Gain  Gain=1/0.03
  Mux : Mux
  Predict : deeplib/Predict  Network=Network from MAT-file  NetworkFunction=squeezenet  NetworkFilePath=D:\Project\GOPS\mdl\RL_model\PPO_1.mat  MiniBatchSize=128  InputDataFormats={ 'input_1', 'UU' }  Predictions=on  Activations={}  ForceInterpretedSim=off  EnableDLNetwork=on  LastKnownNetworkFilePath='D:\Project\GOPS\mdl\RL_model\PPO_1.mat'  LastKnownNetworkTimeStamp=739865.536458333372138440608978271484375
  Rate Transition : RateTransition  OutPortSampleTime=0.01
  Reshape : Reshape  OutputDimensionality=Row vector (2-D)
  Reshape2 : Reshape
  cs : Gain  Gain=-1000
  ks : Gain  Gain=-20000
  F_sus : Outport
  F_ctr : Outport  Port=2
  wires:
  Mux/1 -> Reshape/1
  Reshape/1 -> Rate Transition/1
  a_s/1 -> Gain1/1
  Predict/1 -> Reshape2/1
  Gain1/1 -> Mux/1
  Gain3/1 -> Mux/3
  Constant/1 -> ?
  Constant1/1 -> ?
  Constant2/1 -> ?
  Gain/1 -> F_ctr/1, Add/1
  Reshape2/1 -> Gain/1
  v_def/1 -> cs/1, Gain2/1
  Add1/1 -> Add/2
  cs/1 -> Add1/2
  x_def/1 -> ks/1, Gain3/1
  ks/1 -> Add1/1
  Add/1 -> F_sus/1
  Rate Transition/1 -> Predict/1
  v_s/1 -> Mux/2
  Gain2/1 -> Mux/4

== system RL_sus_quarter_sim/Quarter_sys/Control/Y_1/Realistic Sky-Hook ==
  v_def : Inport
  v_s : Inport  Port=2
  x_def : Inport  Port=3
  Add : Sum  Inputs=+++
  Cs : Gain  Gain=-1500
  Gain : Gain  Gain=-1
  Product1 : Product
  Realistic_C : Constant  Value=500
  ks : Gain  Gain=-20000
  F_sus : Outport
  wires:
  Gain/1 -> Add/1
  Product1/1 -> Gain/1
  Realistic_C/1 -> Product1/2
  v_s/1 -> Product1/1
  x_def/1 -> ks/1
  ks/1 -> Add/2
  Add/1 -> F_sus/1
  v_def/1 -> Cs/1
  Cs/1 -> Add/3

== system RL_sus_quarter_sim/Quarter_sys/Control/Y_1/SH_ADD ==
  x_def : Inport
  v_def : Inport  Port=2
  a_def : Inport  Port=3
  a_s : Inport  Port=4
  v_s : Inport  Port=5
  Add2 : Sum
  Add3 : Sum
  Constant : Constant  Value=1.4*2*pi
  Constant2 : Constant  Value=-1
  Constant3 : Constant
  Delta_C1 : Gain  Gain=500
  Gain1 : Gain  Gain=-1
  Lmbada_C1 : Constant  Value=1000
  MATLAB Function : MATLAB Function  TreatAsAtomicUnit=on
  Product3 : Product
  Switch1 : Switch  Criteria=u2 > Threshold  SaturateOnIntegerOverflow=off  InputSameDT=off
  To Workspace : ToWorkspace  VariableName=FS_result  SampleTime=-1
  ks1 : Gain  Gain=-20000
  F_sus : Outport
  wires:
  Switch1/1 -> Delta_C1/1
  x_def/1 -> ks1/1
  Constant2/1 -> Switch1/3
  v_def/1 -> Product3/1, MATLAB Function/3(vdef)
  Add3/1 -> F_sus/1
  Gain1/1 -> Add3/1
  Add2/1 -> Product3/2
  MATLAB Function/1(y) -> Switch1/2
  Product3/1 -> Gain1/1
  Lmbada_C1/1 -> Add2/2
  Delta_C1/1 -> Add2/1
  ks1/1 -> Add3/2
  Constant3/1 -> Switch1/1
  a_s/1 -> MATLAB Function/1(as)
  v_s/1 -> MATLAB Function/2(vs)
  Constant/1 -> MATLAB Function/4(alpha)
  MATLAB Function/2(FS) -> To Workspace/1

== system RL_sus_quarter_sim/Quarter_sys/Control/Y_1/SH_ADD_modify ==
  x_def : Inport
  v_def : Inport  Port=2
  a_def : Inport  Port=3
  a_s : Inport  Port=4
  v_s : Inport  Port=5
  ADD1 : Subsystem
  Add3 : Sum
  Gain1 : Gain  Gain=-1
  Gain2 : Gain  Gain=2*pi
  MATLAB Function : MATLAB Function  TreatAsAtomicUnit=on
  Modify_SHADD : Subsystem
  Multiport Switch1 : MultiPortSwitch  Inputs=2  SaturateOnIntegerOverflow=off  InputSameDT=off
  Product3 : Product
  SH1 : Subsystem
  alpha1 : Constant  Value=1.41
  cs : Constant  Value=1000
  ks : Constant  Value=20000
  ks1 : Gain  Gain=-20000
  ms : Constant  Value=400
  F_sus : Outport
  wires:
  x_def/1 -> ks1/1
  Add3/1 -> F_sus/1
  Gain1/1 -> Add3/1
  Multiport Switch1/1 -> Product3/2
  Product3/1 -> Gain1/1
  ks1/1 -> Add3/2
  Gain2/1 -> MATLAB Function/3(alpha)
  MATLAB Function/1(y) -> Multiport Switch1/1
  v_def/1 -> SH1/1(v_def), ADD1/1(v_def), Product3/1, MATLAB Function/2(vdef)
  SH1/1(Out1) -> Multiport Switch1/2
  ms/1 -> MATLAB Function/6(ms)
  v_s/1 -> SH1/2(v_s), MATLAB Function/1(vs)
  alpha1/1 -> Gain2/1
  ADD1/1(F_sus1) -> Multiport Switch1/3
  a_s/1 -> ADD1/2(a_s)
  ks/1 -> MATLAB Function/5(ks)
  cs/1 -> MATLAB Function/4(cs)

== system RL_sus_quarter_sim/Quarter_sys/Control/Y_1/SH_ADD_new_FS ==
  x_def : Inport
  v_def : Inport  Port=2
  a_def : Inport  Port=3
  a_s : Inport  Port=4
  v_s : Inport  Port=5
  Add2 : Sum
  Add3 : Sum
  Constant : Constant  Value=1.4*2*pi
  Constant2 : Constant  Value=-1
  Constant3 : Constant
  Delta_C1 : Gain  Gain=500
  Gain1 : Gain  Gain=-1
  Lmbada_C1 : Constant  Value=1000
  MATLAB Function : MATLAB Function  TreatAsAtomicUnit=on
  Modify_SHADD : Subsystem
  Product3 : Product
  Switch1 : Switch  Criteria=u2 > Threshold  SaturateOnIntegerOverflow=off  InputSameDT=off
  ks1 : Gain  Gain=-20000
  F_sus : Outport
  wires:
  Constant/1 -> MATLAB Function/4(alpha)
  v_s/1 -> MATLAB Function/2(vs)
  a_s/1 -> MATLAB Function/1(as)
  Constant3/1 -> Switch1/1
  ks1/1 -> Add3/2
  Delta_C1/1 -> Add2/1
  Lmbada_C1/1 -> Add2/2
  Product3/1 -> Gain1/1
  MATLAB Function/1(y) -> Switch1/2
  Add2/1 -> Product3/2
  Gain1/1 -> Add3/1
  Add3/1 -> F_sus/1
  v_def/1 -> MATLAB Function/3(vdef), Product3/1
  Constant2/1 -> Switch1/3
  x_def/1 -> ks1/1
  Switch1/1 -> Delta_C1/1

== system RL_sus_quarter_sim/Quarter_sys/Control/Y_1/SH_ADD_new_as_as_xdef^2 ==
  x_def : Inport
  v_def : Inport  Port=2
  v_s : Inport  Port=3
  a_s : Inport  Port=4
  a_def : Inport  Port=5
  2nd_FS_adef_vs : Subsystem
  ADD : Subsystem
  SH : Subsystem
  Scope : Scope
      settings: ActiveDisplayYMinimum=-420.62798  ActiveDisplayYMaximum=3660.55556  DataLoggingVariableName=ScopeData19
  Scope1 : Scope
      settings: ActiveDisplayYMinimum=-36.33724  ActiveDisplayYMaximum=1.39762  DataLoggingVariableName=ScopeData21
  Switch1 : Switch  Criteria=u2 > Threshold  SaturateOnIntegerOverflow=off  InputSameDT=off
  F_sus : Outport
  wires:
  a_def/1 -> ?
  Switch1/1 -> F_sus/1
  2nd_FS_adef_vs/1(FS2) -> Switch1/2, Scope/1
  a_s/1 -> 2nd_FS_adef_vs/1(as), ADD/3(a_s)
  SH/1(Out1) -> Switch1/3
  ADD/1(F_sus1) -> Switch1/1
  x_def/1 -> 2nd_FS_adef_vs/2(xdef), ADD/1(x_def), SH/3(x_def), Scope1/1
  v_def/1 -> SH/1(v_def), ADD/2(v_def)
  v_s/1 -> SH/2(v_s)

== system RL_sus_quarter_sim/Quarter_sys/Control/Y_1/SH_ADD_new_as_au_xdef_vdef ==
  x_def : Inport
  v_def : Inport  Port=2
  v_s : Inport  Port=3
  a_s : Inport  Port=4
  a_u : Inport  Port=5
  2nd_FS_adef_vs : Subsystem
  ADD : Subsystem
  SH : Subsystem
  Scope : Scope
      settings: ActiveDisplayYMinimum=-11070.12093  ActiveDisplayYMaximum=35632.12084  DataLoggingVariableName=ScopeData19
  Scope1 : Scope
      settings: ActiveDisplayYMinimum=-36.33724  ActiveDisplayYMaximum=1.39762  DataLoggingVariableName=ScopeData21
  Switch1 : Switch  Criteria=u2 > Threshold  SaturateOnIntegerOverflow=off  InputSameDT=off
  F_sus : Outport
  wires:
  v_s/1 -> SH/2(v_s)
  x_def/1 -> Scope1/1, SH/3(x_def), ADD/1(x_def), 2nd_FS_adef_vs/2(xdef)
  ADD/1(F_sus1) -> Switch1/1
  SH/1(Out1) -> Switch1/3
  a_s/1 -> ADD/3(a_s), 2nd_FS_adef_vs/1(as)
  2nd_FS_adef_vs/1(FS2) -> Scope/1, Switch1/2
  Switch1/1 -> F_sus/1
  a_u/1 -> 2nd_FS_adef_vs/4(au)
  v_def/1 -> 2nd_FS_adef_vs/3(vdef), ADD/2(v_def), SH/1(v_def)

== system RL_sus_quarter_sim/Quarter_sys/Control/Y_1/SH_ADD_new_au_vs ==
  x_def : Inport
  v_def : Inport  Port=2
  v_s : Inport  Port=3
  a_u : Inport  Port=4
  a_s : Inport  Port=5
  2nd_FS : Subsystem
  ADD : Subsystem
  SH : Subsystem
  Switch1 : Switch  Criteria=u2 > Threshold  SaturateOnIntegerOverflow=off  InputSameDT=off
  F_sus : Outport
  wires:
  Switch1/1 -> F_sus/1
  2nd_FS/1(FS2) -> Switch1/2
  a_u/1 -> 2nd_FS/2(au)
  a_s/1 -> ADD/3(a_s)
  v_s/1 -> SH/2(v_s), 2nd_FS/1(vs)
  SH/1(Out1) -> Switch1/3
  ADD/1(F_sus1) -> Switch1/1
  x_def/1 -> ADD/1(x_def), SH/3(x_def)
  v_def/1 -> SH/1(v_def), ADD/2(v_def)
